simulink model "motivacion_deadbeat"  (R2018a)
settings: Solver=VariableStepAuto  StartTime=0.0  StopTime=0.5  RelTol=1e-6
settings Model: Creator=pablo  LastModifiedBy=pablo

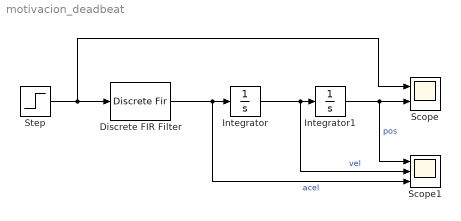
== system motivacion_deadbeat ==
  Discrete FIR Filter : DiscreteFir  Coefficients=[1 -2 1]/(0.1*0.1)  SampleTime=0.1
  Integrator : Integrator
  Integrator1 : Integrator
  Scope : Scope  NumInputPorts=2
  Scope1 : Scope  NumInputPorts=3
  Step : Step  Time=0.1  SampleTime=0
  wires:
  Integrator/1 -> Scope1/2, Integrator1/1  "vel"
  Discrete FIR Filter/1 -> Scope1/3, Integrator/1  "acel"
  Integrator1/1 -> Scope1/1, Scope/2  "pos"
  Step/1 -> Scope/1, Discrete FIR Filter/1
